simulink subsystem "s0519_Better_Lyapunov_maybe"  (R2019b)
settings: Solver=VariableStepAuto  StartTime=0.0  StopTime=10.0  RelTol=1e-3
model mask{k_E=0, k_th=0, k_delta=0, k_ome=0}
undefined symbols (not defined in the file): __PRM__SERIALIZED__DATA__, PARAMS, SubsystemReferenceBlock
settings Model: Creator=francescoceresetti  LastModifiedBy=alessandro

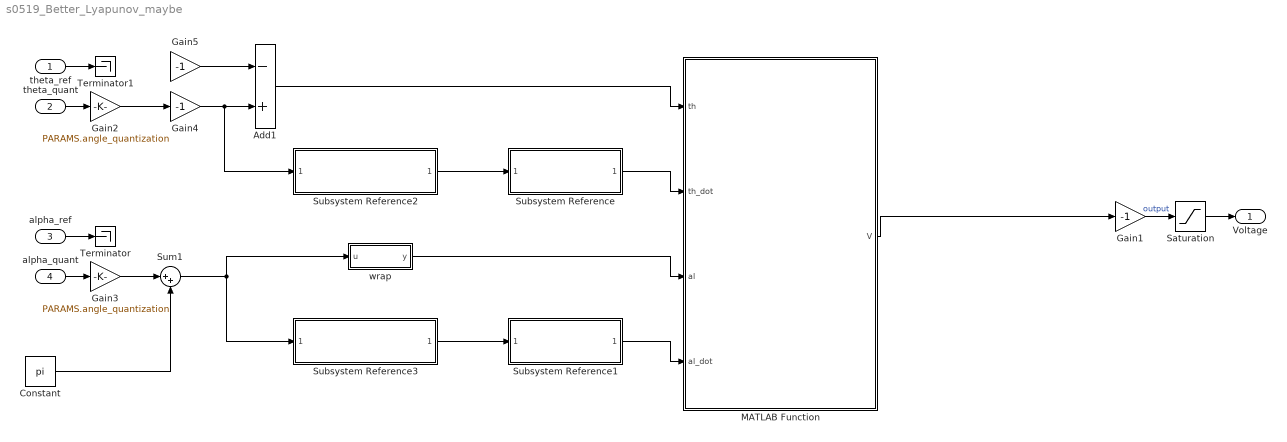
== system s0519_Better_Lyapunov_maybe ==
  theta_ref : Inport
  theta_quant : Inport  Port=2
  alpha_ref : Inport  Port=3
  alpha_quant : Inport  Port=4
  Add1 : Sum  Inputs=-+
  Constant : Constant  Value=pi
  Gain1 : Gain  Gain=-1
  Gain2 : Gain  Gain=PARAMS.angle_quantization
  Gain3 : Gain  Gain=PARAMS.angle_quantization
  Gain4 : Gain  Gain=-1
  Gain5 : Gain  Gain=-1
  MATLAB Function : MATLAB Function  TreatAsAtomicUnit=on
  Saturation : Saturate  UpperLimit=PARAMS.V_sat  LowerLimit=-PARAMS.V_sat
  Subsystem Reference : Subsystem  BlockKeywords=__PRM__SERIALIZED__DATA__:SubsystemReferenceBlock  ReferencedSubsystem=Filtered_Derivative  num=num_der_filter  den=den_der_filter
  Subsystem Reference1 : Subsystem  BlockKeywords=__PRM__SERIALIZED__DATA__:SubsystemReferenceBlock  ReferencedSubsystem=Filtered_Derivative  num=num_der_filter  den=den_der_filter
  Subsystem Reference2 : Subsystem  BlockKeywords=__PRM__SERIALIZED__DATA__:SubsystemReferenceBlock  ReferencedSubsystem=Polynomial_Filter
  Subsystem Reference3 : Subsystem  BlockKeywords=__PRM__SERIALIZED__DATA__:SubsystemReferenceBlock  ReferencedSubsystem=Polynomial_Filter
  Sum1 : Sum  Inputs=|++
  Terminator : Terminator
  Terminator1 : Terminator
  wrap : MATLAB Function  TreatAsAtomicUnit=on
  Voltage : Outport
  wires:
  alpha_quant/1 -> Gain3/1
  Add1/1 -> MATLAB Function/1(th)
  theta_quant/1 -> Gain2/1
  Subsystem Reference1/1 -> MATLAB Function/4(al_dot)
  Subsystem Reference/1 -> MATLAB Function/2(th_dot)
  Gain3/1 -> Sum1/1
  wrap/1(y) -> MATLAB Function/3(al)
  Saturation/1 -> Voltage/1
  Gain4/1 -> Add1/2, Subsystem Reference2/1
  Gain5/1 -> Add1/1
  Gain2/1 -> Gain4/1
  Gain1/1 -> Saturation/1  "output"
  alpha_ref/1 -> Terminator/1
  MATLAB Function/1(V) -> Gain1/1
  Sum1/1 -> wrap/1(u), Subsystem Reference3/1
  Constant/1 -> Sum1/2
  Subsystem Reference3/1 -> Subsystem Reference1/1
  Subsystem Reference2/1 -> Subsystem Reference/1
  theta_ref/1 -> Terminator1/1

== matlab function s0519_Better_Lyapunov_maybe/MATLAB Function ==
  data: th input; V output; th_dot input; al input; al_dot input; PARAMS parameter; k_E parameter; k_ome parameter; k_th parameter; k_delta parameter
function V = fcn(th, th_dot, al, al_dot, PARAMS, k_E, k_ome, k_th, k_delta)
    g = PARAMS.g;

    mp = PARAMS.mp;
    Lp = PARAMS.Lp;
    mr = PARAMS.mr;
    Lr = PARAMS.Lr;
    l1 = PARAMS.l1;
    l2 = PARAMS.l2;
    Jm = PARAMS.Jm;

    Jh = PARAMS.Jh;
    Cal = PARAMS.Cal;
    Cth = PARAMS.Cth;

    K = PARAMS.K;
    
    R = PARAMS.Rm;
    ki = PARAMS.ki;
    kv = PARAMS.kv;



    V = kv*th_dot - (R*(k_th*th + k_delta*th_dot + (144*Lr*k_ome*l2*cos(al)*((mp*sin(2*al)*(Lp^2 + 12*l2^2)*th_dot^2)/24 + g*l2*mp*sin(al)))/(12*Jh*Lp^2 + 12*Jm*Lp^2 + 144*Jh*l2^2 + 144*Jm*l2^2 + 12*Lp^2*Lr^2*mp + Lp^2*Lr^2*mr + 12*Lp^2*l1^2*mr + 144*Lr^2*l2^2*mp + 12*Lr^2*l2^2*mr + 144*l1^2*l2^2*mr + Lp^4*mp*sin(al)^2 + 144*l2^4*mp*sin(al)^2 - 144*Lr^2*l2^2*mp*cos(al)^2 + 24*Lp^2*l2^2*mp*sin(al)^2) - (2*al_dot*k_ome*mp*sin(al)*(Lp^2 + 12*l2^2)*(th_dot*cos(al)*Lp^2 + 12*th_dot*cos(al)*l2^2 + 6*Lr*al_dot*l2))/(12*Jh*Lp^2 + 12*Jm*Lp^2 + 144*Jh*l2^2 + 144*Jm*l2^2 + 12*Lp^2*Lr^2*mp + Lp^2*Lr^2*mr + 12*Lp^2*l1^2*mr + 144*Lr^2*l2^2*mp + 12*Lr^2*l2^2*mr + 144*l1^2*l2^2*mr + Lp^4*mp*sin(al)^2 + 144*l2^4*mp*sin(al)^2 - 144*Lr^2*l2^2*mp*cos(al)^2 + 24*Lp^2*l2^2*mp*sin(al)^2)))/(ki*(k_E*(al_dot*((al_dot*mp*(Lp^2 + 12*l2^2))/24 - (Lr*l2*mp*th_dot*cos(al))/2) + th_dot*((th_dot*(Jh + Jm + Lr^2*mp + (Lr^2*mr)/12 + l1^2*mr - l2^2*mp*(cos(al)^2 - 1) - (Lp^2*mp*(cos(al)^2 - 1))/12))/2 - (Lr*al_dot*l2*mp*cos(al))/2) + g*l2*mp*(cos(al) - 1)) + (12*k_ome*(Lp^2 + 12*l2^2))/(12*Jh*Lp^2 + 12*Jm*Lp^2 + 144*Jh*l2^2 + 144*Jm*l2^2 + 12*Lp^2*Lr^2*mp + Lp^2*Lr^2*mr + 12*Lp^2*l1^2*mr + 144*Lr^2*l2^2*mp + 12*Lr^2*l2^2*mr + 144*l1^2*l2^2*mr + Lp^4*mp*sin(al)^2 + 144*l2^4*mp*sin(al)^2 - 144*Lr^2*l2^2*mp*cos(al)^2 + 24*Lp^2*l2^2*mp*sin(al)^2)));

end

== matlab function s0519_Better_Lyapunov_maybe/wrap ==
  data: u input; y output
function y = wrap(u)
stop_condition = false;
y = u;
while ~stop_condition
    if y > pi
        y = y - 2*pi;
    elseif y < -pi
        y = y + 2*pi;
    else
        stop_condition = true;
    end
end
